simulink model "test_IO_log_test"  (R2018b)
settings: Solver=VariableStepAuto  StartTime=0.0  StopTime=10.0  RelTol=1e-3
libraries: test_IO_log_lib x1
settings Model: Creator=taylorreynolds  LastModifiedBy=Taylor

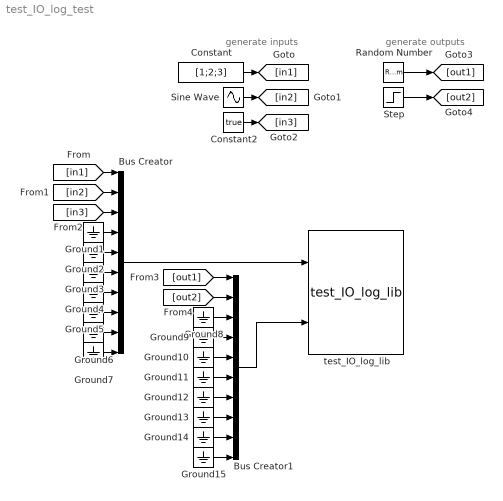
== system test_IO_log_test ==
  note: generate inputs
  note: generate outputs
  Bus Creator : BusCreator  Inputs=10
  Bus Creator1 : BusCreator  Inputs=10
  Constant : Constant  Value=[1;2;3]  OutDataTypeStr=int32  LockScale=on
  Constant2 : Constant  Value=true  OutDataTypeStr=boolean
  Ground{1..15} (15 alike) : Ground
  Random Number : RandomNumber  SampleTime=0.1
  Sine Wave : Sin  SampleTime=0
  Step : Step  Time=[1,1]  Before=[0,0]  After=[1,2]  SampleTime=0
  test_IO_log_lib : test_IO_log_lib/test_IO_log_lib  iString1="\"input_name1\""  iString2="\"input_name2\""  iString3="\"input_name3\""  iString4="\"ignore\""  iString5="\"ignore\""  iString6="\"ignore\""  iString7="\"ignore\""  iString8="\"ignore\""  iString9="\"ignore\""  iString10="\"ignore\""  oString1="\"output_name1\""  oString2="\"output_name2\""  oString3="\"ignore\""  oString4="\"ignore\""  oString5="\"ignore\""  oString6="\"ignore\""  oString7="\"ignore\""  oString8="\"ignore\""  oString9="\"ignore\""  oString10="\"ignore\""
  wires:
  Constant/1 -> [in1]
  Random Number/1 -> [out1]
  Bus Creator/1 -> test_IO_log_lib/1
  Sine Wave/1 -> [in2]
  [in3] -> Bus Creator/3
  Bus Creator1/1 -> test_IO_log_lib/2
  Step/1 -> [out2]
  Ground1/1 -> Bus Creator/4
  Ground2/1 -> Bus Creator/5
  Ground3/1 -> Bus Creator/6
  Ground4/1 -> Bus Creator/7
  Ground5/1 -> Bus Creator/8
  Ground6/1 -> Bus Creator/9
  Ground7/1 -> Bus Creator/10
  Constant2/1 -> [in3]
  [in1] -> Bus Creator/1
  [in2] -> Bus Creator/2
  [out1] -> Bus Creator1/1
  [out2] -> Bus Creator1/2
  Ground8/1 -> Bus Creator1/3
  Ground9/1 -> Bus Creator1/4
  Ground10/1 -> Bus Creator1/5
  Ground11/1 -> Bus Creator1/6
  Ground12/1 -> Bus Creator1/7
  Ground13/1 -> Bus Creator1/8
  Ground14/1 -> Bus Creator1/9
  Ground15/1 -> Bus Creator1/10
